simulink model "First_order_RC_low_pass_filter"  (R2024b)
settings: Solver=FixedStepAuto  StartTime=0.0  StopTime=100  FixedStep=1e-4  RelTol=1e-3
values from neighbouring files (symbols this model uses):
  RC = 0.001    [run_First_order_RC_low_pass_filter.m]
settings Model: Creator=sajim  LastModifiedBy=sajim

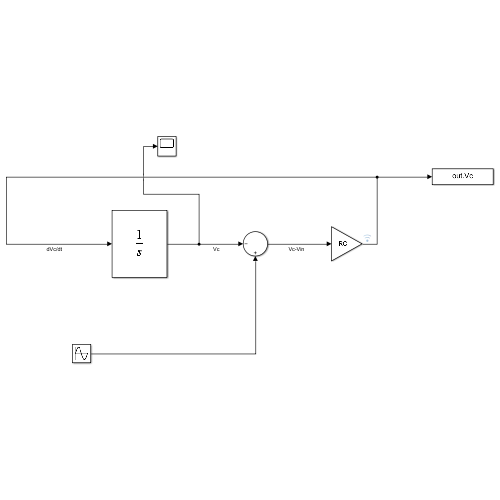
[thumbnail: Simulink's stored preview of the top-level diagram]
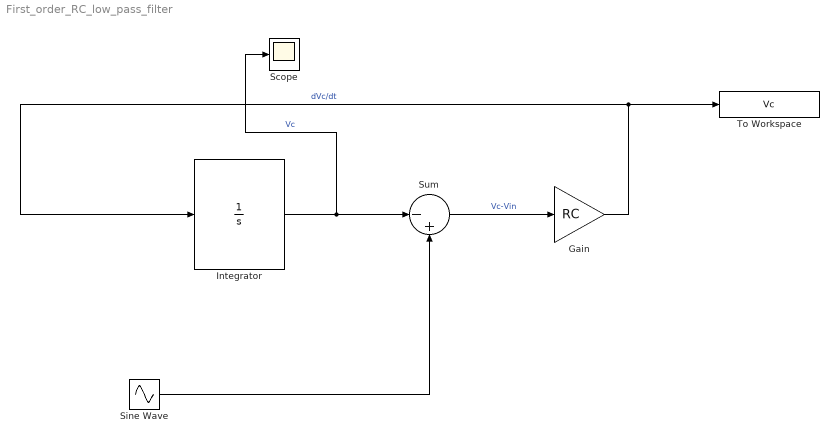
== system First_order_RC_low_pass_filter ==
  Gain : Gain  Gain=RC
  Integrator : Integrator  InitialCondition=0.01
  Scope : Scope
  Sine Wave : Sin  Amplitude=5  Frequency=0.05  SampleTime=0
  Sum : Sum  Inputs=|-+
  To Workspace : ToWorkspace  VariableName=Vc  SaveFormat=Timeseries  SampleTime=-1
  wires:
  Integrator/1 -> Scope/1, Sum/1  "Vc"
  Sum/1 -> Gain/1  "Vc-Vin"
  Sine Wave/1 -> Sum/2
  Gain/1 -> Integrator/1, To Workspace/1  "dVc/dt"
